simulink model "Factorial_FOR_WHILE_MATLAB"  (R2021a)
settings: Solver=FixedStepDiscrete  StartTime=0.0  StopTime=10  RelTol=1e-3
settings Model: Creator=hp  LastModifiedBy=hp
settings OptimizationCC: DefaultParameterBehavior=Inlined  EnhancedBackFolding=on  PassReuseOutputArgsAs=Individual arguments  ZeroExternalMemoryAtStartup=off  ZeroInternalMemoryAtStartup=off  OptimizeBlockOrder=speed  DifferentSizesBufferReuse=on  OptimizationCustomize=off  EfficientTunableParamExpr=on
settings DebuggingCC: ParameterTunabilityLossMsg=error
settings SFSimCC: MATLABDynamicMemAlloc=off
settings RTWCC: SystemTargetFile=ert.tlc  GenCodeOnly=on  TemplateMakefile=ert_default_tmf  GenerateReport=on  IncludeHyperlinkInReport=on  LaunchReport=on  GenerateTraceInfo=on
settings CodeAppCC: ForceParamTrailComments=on  IgnoreCustomStorageClasses=off  OperatorAnnotations=on  SimulinkDataObjDesc=on  SFDataObjDesc=on  InsertBlockDesc=on
settings ERTTargetCC: TargetLangStandard=C99 (ISO)  GenerateSampleERTMain=on  SupportNonFinite=off  SupportComplex=off  InlinedParameterPlacement=NonHierarchical  ERTCustomFileTemplate=example_file_process.tlc  IndentSize=4  EnableUserReplacementTypes=on

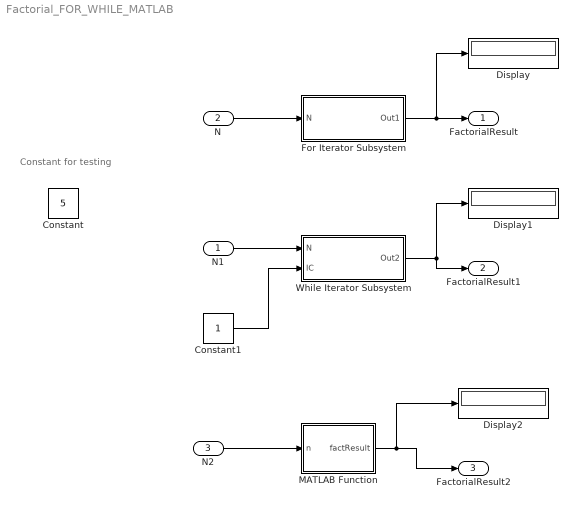
== system Factorial_FOR_WHILE_MATLAB ==
  note: Constant for testing
  N1 : Inport
  N : Inport  Port=2
  N2 : Inport  Port=3
  Constant : Constant  Value=5
  Constant1 : Constant
  Display : Display
  Display1 : Display
  Display2 : Display
  For Iterator Subsystem : Subsystem  TreatAsAtomicUnit=on
  MATLAB Function : MATLAB Function  TreatAsAtomicUnit=on
  While Iterator Subsystem : Subsystem  TreatAsAtomicUnit=on
  FactorialResult : Outport
  FactorialResult1 : Outport  Port=2
  FactorialResult2 : Outport  Port=3
  wires:
  For Iterator Subsystem/1(Out1) -> Display/1, FactorialResult/1
  While Iterator Subsystem/1(Out2) -> FactorialResult1/1, Display1/1
  Constant1/1 -> While Iterator Subsystem/2(IC)
  N1/1 -> While Iterator Subsystem/1(N)
  N/1 -> For Iterator Subsystem/1(N)
  N2/1 -> MATLAB Function/1(n)
  MATLAB Function/1(factResult) -> Display2/1, FactorialResult2/1

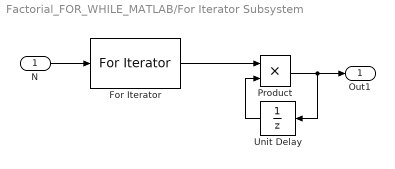
== system Factorial_FOR_WHILE_MATLAB/For Iterator Subsystem ==
  N : Inport
  For Iterator : ForIterator  ResetStates=reset  IterationSource=external
  Product : Product  OutDataTypeStr=uint32
  Unit Delay : UnitDelay  InitialCondition=1  SampleTime=-1  HasFrameUpgradeWarning=on
  Out1 : Outport
  wires:
  N/1 -> For Iterator/1
  For Iterator/1 -> Product/1
  Product/1 -> Unit Delay/1, Out1/1
  Unit Delay/1 -> Product/2

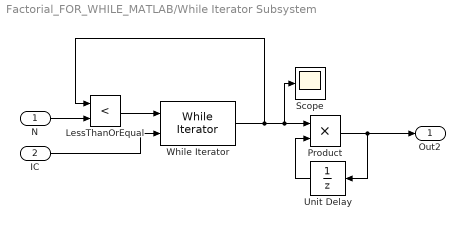
== system Factorial_FOR_WHILE_MATLAB/While Iterator Subsystem ==
  N : Inport
  IC : Inport  Port=2
  LessThanOrEqual : RelationalOperator  Operator=<  OutDataTypeStr=boolean  RndMeth=Simplest
  Product : Product  OutDataTypeStr=uint32
  Scope : Scope
  Unit Delay : UnitDelay  InitialCondition=1  SampleTime=-1  HasFrameUpgradeWarning=on
  While Iterator : WhileIterator  MaxIters=-1  ResetStates=reset  ShowIterationPort=on
  Out2 : Outport
  wires:
  Unit Delay/1 -> Product/2
  Product/1 -> Unit Delay/1, Out2/1
  LessThanOrEqual/1 -> While Iterator/1
  IC/1 -> While Iterator/2
  While Iterator/1 -> LessThanOrEqual/1, Scope/1, Product/1
  N/1 -> LessThanOrEqual/2

== matlab function Factorial_FOR_WHILE_MATLAB/MATLAB Function ==
  data: n input; factResult output
function factResult = fcn(n)

factResult = factorial(n);
